simulink model "boost_shema"  (R2022b)
settings: Solver=FixedStepAuto  StartTime=0.0  StopTime=0.15  FixedStep=2e-8  RelTol=1e-3
undefined symbols (not defined in the file): promena_ref, ref_V, sigbuilder_block, wpref
libraries: spsMeanLib x2, spsSeriesRLCBranchLib x2, spsControlledVoltageSourceLib x1, spsCurrentMeasurementLib x1, spsDiodeLib x1, spsGroundLib x1, cstblocks x1, spsMosfetLib x1, eePwmGenerator x1, spsVariableResistorLib x1, spsVoltageMeasurementLib x1, sps_lib x1
settings Model: SimulationMode=accelerator  Creator=user  LastModifiedBy=user

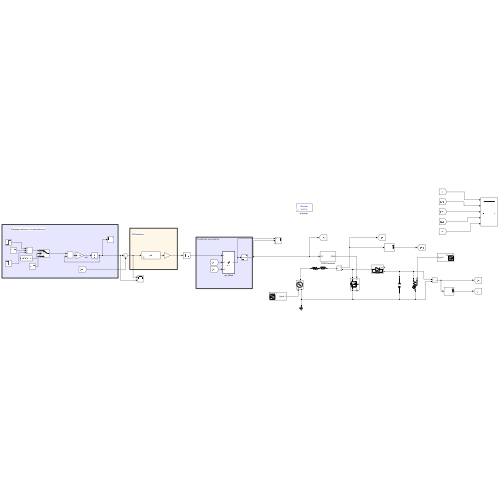
[thumbnail: Simulink's stored preview of the top-level diagram]
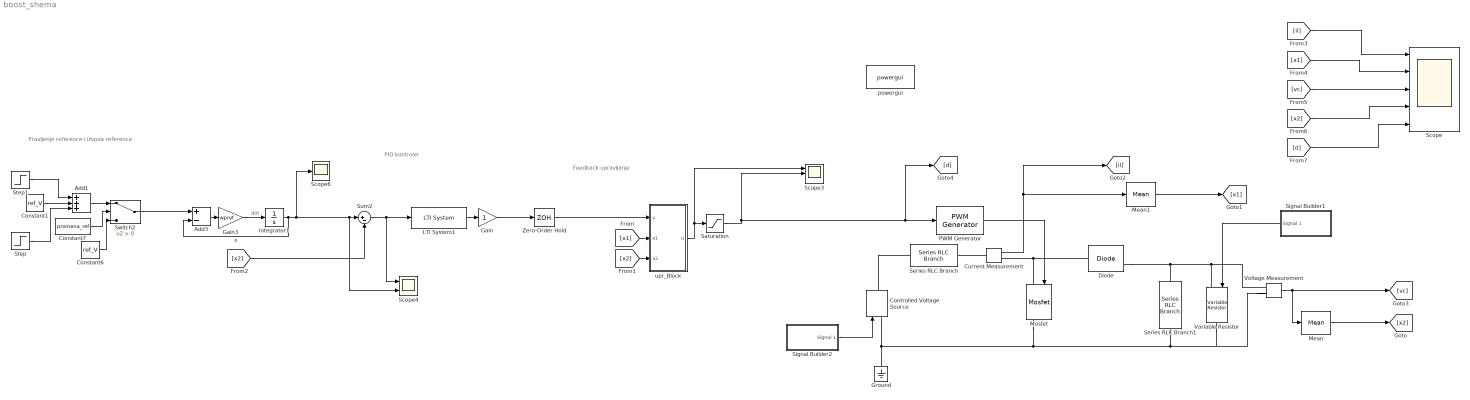
== system boost_shema ==
  note: Pravljenje reference i izvoda reference
  note: PID kontroler
  note: Feedback upravljanje
  Add1 : Sum  Inputs=+++
  Add3 : Sum  Inputs=+-
  Constant1 : Constant  Value=ref_V  SampleTime=-1
  Constant6 : Constant  Value=ref_V  SampleTime=-1
  Constant7 : Constant  Value=promena_ref
  Controlled Voltage Source : spsControlledVoltageSourceLib/Controlled Voltage Source  Initialize=on  Source_Type=AC  Amplitude=0  Phase=0  Frequency=0  Measurements=None
  Current Measurement : spsCurrentMeasurementLib/Current Measurement  PhasorSimulation=off  OutputType=Complex  PSBequivalent=0
  Diode : spsDiodeLib/Diode  Ron=0.5  Lon=0  Vf=0.7  IC=0  UseSnubber=0  Rs=500  Cs=250e-9  Measurements=on
  Gain : Gain
  Gain3 : Gain  Gain=wpref
  Ground : spsGroundLib/Ground  LConnTagsString=a
  Integrator1 : Integrator  InitialCondition=16
  LTI System1 : cstblocks/LTI System  sys=pid  IC=[]
  Mean : spsMeanLib/Mean  Freq=5e4  Vinit=0  Ts=1e-6
  Mean1 : spsMeanLib/Mean  Freq=5e4  Vinit=0  Ts=1e-6
  Mosfet : spsMosfetLib/Mosfet  Ron=0.3  Lon=0  Rd=0.01  Vfd=0  IC=0  Rs=1e5  Cs=inf  Measurements=on
  PWM Generator : eePwmGenerator/PWM Generator  CarrCount=Up  Tper=2e-5  Tdelay=0  Ts=2e-8
  Saturation : Saturate  UpperLimit=1  LowerLimit=0
  Scope : Scope  NumInputPorts=5
  Scope3 : Scope  NumInputPorts=3
  Scope4 : Scope  NumInputPorts=2
  Scope6 : Scope
  Series RLC Branch : spsSeriesRLCBranchLib/Series RLC Branch  LConnTagsString=__new0  RConnTagsString=__new0  BranchType=RL  Resistance=0.2  Inductance=250e-6  SetiL0=off  InitialCurrent=0  Capacitance=1e-6  Setx0=off  InitialVoltage=0  Measurements=None
  Series RLC Branch1 : spsSeriesRLCBranchLib/Series RLC Branch  LConnTagsString=__new0  RConnTagsString=__new0  BranchType=C  Resistance=1  Inductance=250e-6  SetiL0=off  InitialCurrent=0  Capacitance=500e-6  Setx0=off  InitialVoltage=0  Measurements=None
  Signal Builder1 : Subsystem  Tag=STV Subsys  LoadFcn=sigbuilder_block('load');  StartFcn=sigbuilder_block('start');  StopFcn=sigbuilder_block('stop');  ClipboardFcn=sigbuilder_block('clipboard');  mask(Sigbuilder block){tuvar=[0:10]}
      mask help: Simulink:masks:SigbuilderBlock_MD
      mask init:
      | if ~strcmp(get_param(bdroot(gcbh),'SimulationStatus'),'stopped') tuvar = sigbuilder_block('maskInit'); end
      settings: CopyFcn=sigbuilder_block('copy');  DeleteFcn=sigbuilder_block('delete');  ModelCloseFcn=sigbuilder_block('modelClose');  PreSaveFcn=sigbuilder_block('preSave');  PauseFcn=sigbuilder_block('pause');  ContinueFcn=sigbuilder_block('continue');  NameChangeFcn=sigbuilder_block('namechange');  OpenFcn=sigbuilder_block('open',[5.4 30 1141.2 522.6 ]);  CloseFcn=sigbuilder_block('close');
      mask Display: plot(0, 0, 100, 100,[2, 2, 32, 32, 2], [68, 8, 8, 68, 68],[32, 2], [38, 38], [32, 19, 2],[53, 60, 44], [32, 17, 17, 2],[16, 16, 31, 31]);txt = getActiveGroup(gcbh);text(2, 100, txt,'verticalAlignment', 'top');
  Signal Builder2 : Subsystem  Tag=STV Subsys  LoadFcn=sigbuilder_block('load',[5.4 30 1141.2 522.6 ]);  StartFcn=sigbuilder_block('start');  StopFcn=sigbuilder_block('stop');  ClipboardFcn=sigbuilder_block('clipboard');  mask(Sigbuilder block){tuvar=[0:10]}
      mask help: Simulink:masks:SigbuilderBlock_MD
      mask init:
      | if ~strcmp(get_param(bdroot(gcbh),'SimulationStatus'),'stopped') tuvar = sigbuilder_block('maskInit'); end
      settings: CopyFcn=sigbuilder_block('copy');  DeleteFcn=sigbuilder_block('delete');  ModelCloseFcn=sigbuilder_block('modelClose');  PreSaveFcn=sigbuilder_block('preSave');  PauseFcn=sigbuilder_block('pause');  ContinueFcn=sigbuilder_block('continue');  NameChangeFcn=sigbuilder_block('namechange');  OpenFcn=sigbuilder_block('open',[5.4 30 1141.2 522.6 ]);  CloseFcn=sigbuilder_block('close');
      mask Display: plot(0, 0, 100, 100,[2, 2, 32, 32, 2], [68, 8, 8, 68, 68],[32, 2], [38, 38], [32, 19, 2],[53, 60, 44], [32, 17, 17, 2],[16, 16, 31, 31]);txt = getActiveGroup(gcbh);text(2, 100, txt,'verticalAlignment', 'top');
  Step : Step  Time=2  After=-2
  Step1 : Step  Time=1.5  SampleTime=0
  Sum2 : Sum  Inputs=|+-
  Switch2 : Switch  Criteria=u2 > Threshold  SaturateOnIntegerOverflow=off  InputSameDT=off
  Variable Resistor : spsVariableResistorLib/Variable Resistor  Rabsmin=1
      settings: LibrarySourceBlock=sps_lib/Passives/Variable Resistor
  Voltage Measurement : spsVoltageMeasurementLib/Voltage Measurement  PhasorSimulation=off  OutputType=Complex  PSBequivalent=0
  Zero-Order Hold : ZeroOrderHold  SampleTime=1e-5
  powergui : sps_lib/powergui  Priority=1  SimulationMode=Discrete  SampleTime=1e-7  frequency=60  Iterations=50  frequencyindice=0  Pbase=100e6  ErrMax=1e-4  UnitsV=kV  UnitsW=MW  buscounter=0  FunctionMessages=off  echomessages=off  EnableUseOfTLC=off  CurrentSourceSwitches=off  DisableSnubberDevices=off  DisableRonSwitches=off  DisableVfSwitches=off  DisplayEquations=off  AutomaticDiscreteSolvers=off  SolverType=Tustin/Backward Euler (TBE)  Interpol=off  ExternalGateDelay=off  methode=off  Ts=100  x0status=blocks  SPID=on  SwTol=0  HookPort=off  NonlinearTolerance=1e-4  nMaxIteration=100  ContinueOnMaxIteration=off  RestoreLinks=warning  ResistiveCurrentMeasurement=off  Frange=[0:2:500]  Ylog=off  Xlog=on  ShowGrid=off  save=off  variable=ZData  structure=0  ZoomFFT=off  StartTime=0.0  cycles=1  DisplayStyle=1  fundamental=60  FreqAxis=off  MaxFrequency=1000  frequencyindicesteady=1  RmsSteady=1  display=off
  upr_Block : MATLAB Function  TreatAsAtomicUnit=on  SystemSampleTime=1e-5
  wires:
  Voltage Measurement/1 -> [vc], Mean/1
  Saturation/1 -> Scope3/2, [d], PWM Generator/1
  PWM Generator/1 -> Mosfet/1
  Current Measurement/1 -> [il], Mean1/1
  Mean/1 -> [x2]
  Mean1/1 -> [x1]
  Sum2/1 -> LTI System1/1, Scope4/1
  LTI System1/1 -> Gain/1
  [x2] -> Sum2/2
  [x1] -> upr_Block/2(x1)
  Step/1 -> Add1/3
  Gain3/1 -> Integrator1/1  "dot"
  Integrator1/1 -> Add3/2, Scope6/1, Scope4/2, Sum2/1  "R"
  Switch2/1 -> Add3/1
  Gain/1 -> Zero-Order Hold/1
  upr_Block/1(u) -> Scope3/1, Saturation/1
  [x2] -> upr_Block/3(x2)
  Step1/1 -> Add1/1
  Constant7/1 -> Switch2/2
  Constant6/1 -> Switch2/3
  Add1/1 -> Switch2/1
  Add3/1 -> Gain3/1
  Constant1/1 -> Add1/2
  [il] -> Scope/1
  [x1] -> Scope/2
  [vc] -> Scope/3
  [x2] -> Scope/4
  [d] -> Scope/5
  Zero-Order Hold/1 -> upr_Block/1(v)
  Signal Builder2/1(Signal 1) -> Controlled Voltage Source/1
  Signal Builder1/1(Signal 1) -> Variable Resistor/1
  connections:
  Series RLC Branch/LConn1 -- Controlled Voltage Source/RConn1
  Mosfet/LConn1 -- Current Measurement/RConn1 -- Diode/LConn1
  Ground/LConn1 -- Controlled Voltage Source/LConn1 -- Variable Resistor/RConn1 -- Voltage Measurement/LConn2 -- Series RLC Branch1/RConn1 -- Mosfet/RConn1
  Series RLC Branch1/LConn1 -- Voltage Measurement/LConn1 -- Variable Resistor/LConn1 -- Diode/RConn1
  Current Measurement/LConn1 -- Series RLC Branch/RConn1

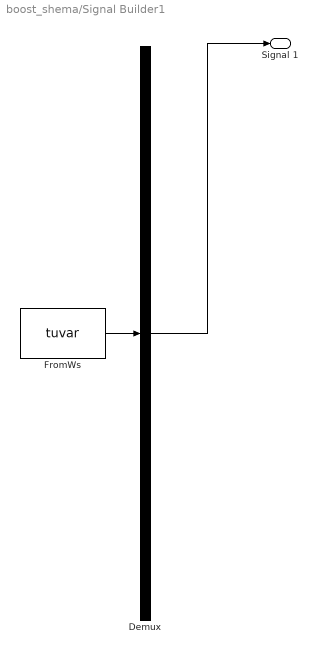
== system boost_shema/Signal Builder1 ==
  Demux : Demux  Tag=STV Demux  Outputs=1
      settings: DisplayOption=none
  FromWs : FromWorkspace  Tag=STV FromWs  VariableName=tuvar
      SigBuilderData=|
      | common.afterFinalStr = 'Extrapolate'
      | common.sampleTime = 0
      | dataSet.timeRange = [0 1]
      | dataSet.name = 'Group 1'
      | sbobj.Groups.Name = 'Group 1'
      | sbobj.Groups.Signals.Name = 'Signal 1'
      | sbobj.Groups.Signals.XData = [0 0.1 0.1 0.2 0.2 0.3 0.3 1]
      | sbobj.Groups.Signals.YData = [15 15 13.5 13.5 16.5 16.5 15 15]
      | sbobj.Groups.TimeRange = [0 1]
  Signal 1 : Outport  Tag=STV Outport
  wires:
  FromWs/1 -> Demux/1
  Demux/1 -> Signal 1/1

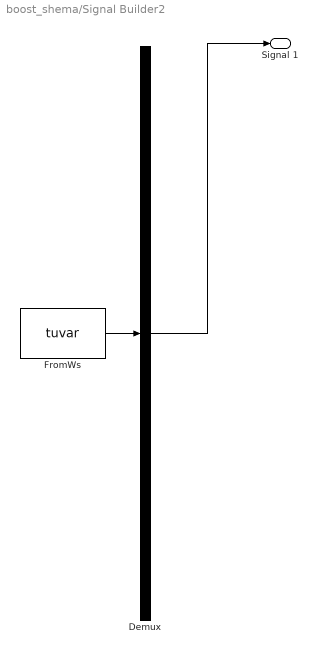
== system boost_shema/Signal Builder2 ==
  Demux : Demux  Tag=STV Demux  Outputs=1
      settings: DisplayOption=none
  FromWs : FromWorkspace  Tag=STV FromWs  VariableName=tuvar
      SigBuilderData=|
      | common.afterFinalStr = 'Extrapolate'
      | common.sampleTime = 0
      | dataSet.timeRange = [0 1]
      | dataSet.name = 'Group 1'
      | sbobj.Groups.Name = 'Group 1'
      | sbobj.Groups.Signals.Name = 'Signal 1'
      | sbobj.Groups.Signals.XData = [0 0.2 0.2 0.3 0.3 0.375 0.375 1]
      | sbobj.Groups.Signals.YData = [12 12 13 13 11 11 12 12]
      | sbobj.Groups.TimeRange = [0 1]
  Signal 1 : Outport  Tag=STV Outport
  wires:
  Demux/1 -> Signal 1/1
  FromWs/1 -> Demux/1

== matlab function boost_shema/upr_Block ==
  data: v input; u output; x1 input; x2 input
function u  = fcn(v,x1,x2)
u = (v/2000-x1+x2/15)/x1;

end
